simulink model "highPass_filter"  (R2020a)
settings: Solver=VariableStepAuto  StartTime=0.0  StopTime=10.0  RelTol=1e-3
model workspace (MAT data in the model file):
  gainA = 0.5792
  gainB = 0.1584
settings Model: Creator=INDRAJIT MARATHE  LastModifiedBy=INDRAJIT MARATHE

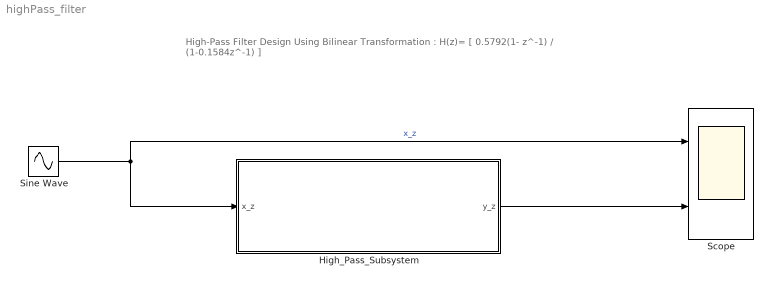
== system highPass_filter ==
  note: High-Pass Filter Design Using Bilinear Transformation :
      |
      | H(z)= [ 0.5792(1- z^-1) / (1-0.1584z^-1) ]
  High_Pass_Subsystem : Subsystem
  Scope : Scope  NumInputPorts=2
  Sine Wave : Sin  Frequency=600  SampleTime=0
  wires:
  Sine Wave/1 -> High_Pass_Subsystem/1(x_z), Scope/1  "x_z"
  High_Pass_Subsystem/1(y_z) -> Scope/2

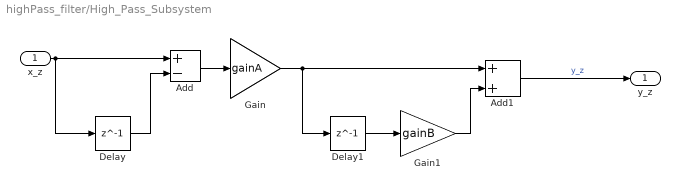
== system highPass_filter/High_Pass_Subsystem ==
  x_z : Inport
  Add : Sum  Inputs=+-
  Add1 : Sum
  Delay : Delay  DelayLength=1
  Delay1 : Delay  DelayLength=1
  Gain : Gain  Gain=gainA
  Gain1 : Gain  Gain=gainB
  y_z : Outport
  wires:
  Gain/1 -> Add1/1, Delay1/1
  Add/1 -> Gain/1
  Delay/1 -> Add/2
  x_z/1 -> Add/1, Delay/1
  Delay1/1 -> Gain1/1
  Add1/1 -> y_z/1  "y_z"
  Gain1/1 -> Add1/2
